simulink model "to_tank_system_2_2015a"  (R2015a)
settings: Solver=ode1  StartTime=0.0  StopTime=runtime  FixedStep=0.01  RelTol=1e-3
values from neighbouring files (symbols this model uses):
  A_1 = 10    [main.m]
  A_2 = 5    [main.m]
  H = 1    [main.m]
  k_2 = 5    [main.m]
  k_3 = 2    [main.m]
  k_i = 0.9    [main.m]
  k_p = 8.3    [main.m]
  noise = 0    [main.m]
  ro = 1    [main.m]
  time_delay = 0.01    [main.m]
  w_1_max = 1000    [main.m]
settings Model: Creator=Sondre  LastModifiedBy=Sondre

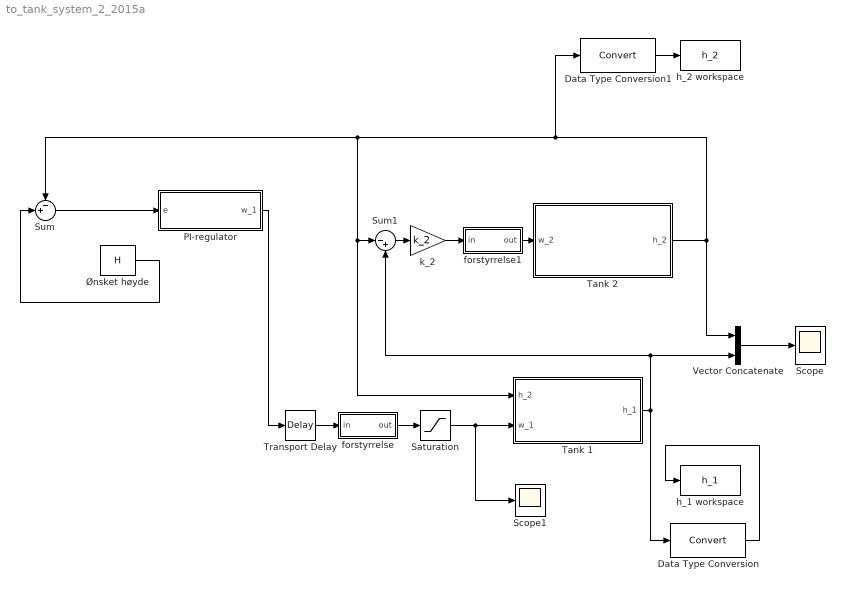
== system to_tank_system_2_2015a ==
  Data Type Conversion : DataTypeConversion
  Data Type Conversion1 : DataTypeConversion
  PI-regulator : Subsystem
  Saturation : Saturate  UpperLimit=w_1_max  LowerLimit=0
  Scope : Scope
      settings: TimeRange=auto  LimitDataPoints=on  MaxDataPoints=5000  SaveToWorkspace=off  SaveName=ScopeData  YMin=-0.19051  YMax=1.71461  SampleTime=-1  DataFormat=Array
  Scope1 : Scope
      settings: TimeRange=auto  MaxDataPoints=5000  SaveToWorkspace=off  YMin=-0.5  YMax=4.5  SampleTime=-1
  Sum : Sum  Inputs=-+|
  Sum1 : Sum  Inputs=|-+
  Tank 1 : Subsystem
  Tank 2 : Subsystem
  Transport Delay : TransportDelay  DelayTime=time_delay
  Vector Concatenate : Concatenate
  forstyrrelse : Subsystem
  forstyrrelse1 : Subsystem
  h_1 workspace : ToWorkspace  VariableName=h_1  SaveFormat=Timeseries  SampleTime=-1
  h_2 workspace : ToWorkspace  VariableName=h_2  SaveFormat=Timeseries  SampleTime=-1
  k_2 : Gain  Gain=k_2
  Ønsket høyde : Constant  Value=H
  wires:
  Tank 2/1(h_2) -> Sum1/1, Tank 1/1(h_2), Sum/1, Data Type Conversion1/1, Vector Concatenate/1
  Sum1/1 -> k_2/1
  Tank 1/1(h_1) -> Data Type Conversion/1, Sum1/2, Vector Concatenate/2
  Vector Concatenate/1 -> Scope/1
  Ønsket høyde/1 -> Sum/2
  Saturation/1 -> Scope1/1, Tank 1/2(w_1)
  Sum/1 -> PI-regulator/1(e)
  forstyrrelse/1(out) -> Saturation/1
  k_2/1 -> forstyrrelse1/1(in)
  forstyrrelse1/1(out) -> Tank 2/1(w_2)
  PI-regulator/1(w_1) -> Transport Delay/1
  Transport Delay/1 -> forstyrrelse/1(in)
  Data Type Conversion/1 -> h_1 workspace/1
  Data Type Conversion1/1 -> h_2 workspace/1

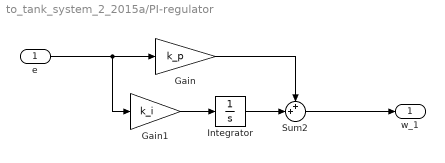
== system to_tank_system_2_2015a/PI-regulator ==
  e : Inport
  Gain : Gain  Gain=k_p
  Gain1 : Gain  Gain=k_i
  Integrator : Integrator
  Sum2 : Sum  Inputs=++|
  w_1 : Outport
  wires:
  Integrator/1 -> Sum2/2
  Gain/1 -> Sum2/1
  Gain1/1 -> Integrator/1
  e/1 -> Gain1/1, Gain/1
  Sum2/1 -> w_1/1

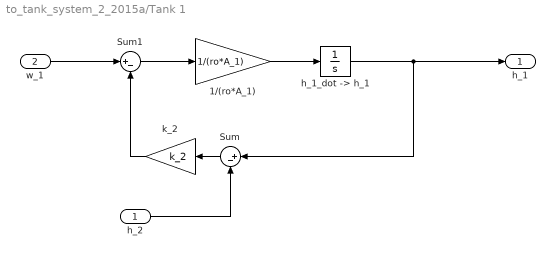
== system to_tank_system_2_2015a/Tank 1 ==
  h_2 : Inport
  w_1 : Inport  Port=2
  1/(ro*A_1) : Gain  Gain=1/(ro*A_1)
  Sum : Sum  Inputs=|+-
  Sum1 : Sum  Inputs=|+-
  "h_1_dot -> h_1" : Integrator
  k_2 : Gain  Gain=k_2
  h_1 : Outport
  wires:
  "h_1_dot -> h_1"/1 -> h_1/1, Sum/1
  Sum1/1 -> 1/(ro*A_1)/1
  h_2/1 -> Sum/2
  w_1/1 -> Sum1/1
  Sum/1 -> k_2/1
  1/(ro*A_1)/1 -> "h_1_dot -> h_1"/1
  k_2/1 -> Sum1/2

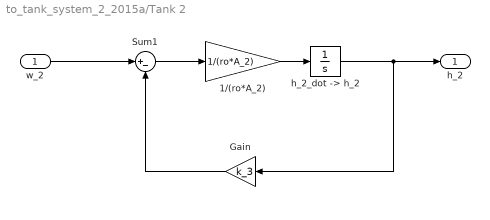
== system to_tank_system_2_2015a/Tank 2 ==
  w_2 : Inport
  1/(ro*A_2) : Gain  Gain=1/(ro*A_2)
  Gain : Gain  Gain=k_3
  Sum1 : Sum  Inputs=|+-
  "h_2_dot -> h_2" : Integrator
  h_2 : Outport
  wires:
  Gain/1 -> Sum1/2
  w_2/1 -> Sum1/1
  Sum1/1 -> 1/(ro*A_2)/1
  1/(ro*A_2)/1 -> "h_2_dot -> h_2"/1
  "h_2_dot -> h_2"/1 -> h_2/1, Gain/1

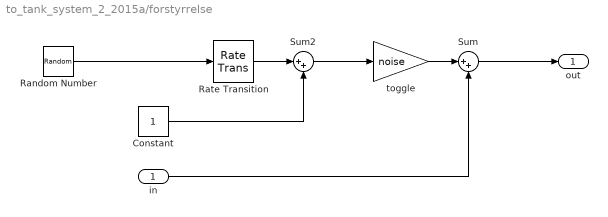
== system to_tank_system_2_2015a/forstyrrelse ==
  in : Inport
  Constant : Constant
  Random Number : RandomNumber  SampleTime=0.1
  Rate Transition : RateTransition
  Sum : Sum  Inputs=|++
  Sum2 : Sum  Inputs=|++
  toggle : Gain  Gain=noise
  out : Outport
  wires:
  Rate Transition/1 -> Sum2/1
  Random Number/1 -> Rate Transition/1
  Constant/1 -> Sum2/2
  in/1 -> Sum/2
  Sum/1 -> out/1
  toggle/1 -> Sum/1
  Sum2/1 -> toggle/1

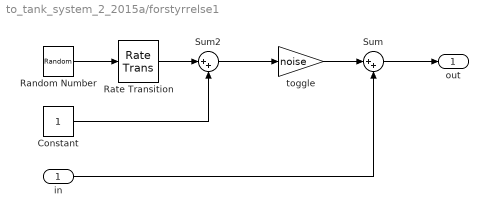
== system to_tank_system_2_2015a/forstyrrelse1 ==
  in : Inport
  Constant : Constant
  Random Number : RandomNumber  SampleTime=0.1
  Rate Transition : RateTransition
  Sum : Sum  Inputs=|++
  Sum2 : Sum  Inputs=|++
  toggle : Gain  Gain=noise
  out : Outport
  wires:
  Rate Transition/1 -> Sum2/1
  Random Number/1 -> Rate Transition/1
  Constant/1 -> Sum2/2
  in/1 -> Sum/2
  Sum/1 -> out/1
  toggle/1 -> Sum/1
  Sum2/1 -> toggle/1
